simulink model "LQR_spring_2mass_damper_system"  (R2022b)
settings: Solver=FixedStepAuto  StartTime=0  StopTime=Tf  FixedStep=dt  RelTol=1e-3
values from neighbouring files (symbols this model uses):
  A = [0 1 0 0; -(k1+k2)/m1 -(c1+c2)/m1 k2/m1 c2/m1;0 0 0 1;k2/m2 c2/m2 -k2/m2 -c2/m2]    [LQR_2mass__slx_main.m]
  B = [0 0;1/m1 0;0 0;0 1/m2]    [LQR_2mass__slx_main.m]
  c1 = 1    [LQR_2mass__slx_main.m]
  c2 = 2    [LQR_2mass__slx_main.m]
  control_on = true    [LQR_2mass__slx_main.m]
  control_period = 0.1    [LQR_2mass__slx_main.m]
  K = inv(R)*B'*P    [LQR_2mass__slx_main.m]
  k1 = 10    [LQR_2mass__slx_main.m]
  k2 = 20    [LQR_2mass__slx_main.m]
  m1 = 1    [LQR_2mass__slx_main.m]
  m2 = 5    [LQR_2mass__slx_main.m]
  r = [0 0 0 0]'    [LQR_2mass__slx_main.m]
  v1 = 0    [LQR_2mass__slx_main.m]
  v2 = 0    [LQR_2mass__slx_main.m]
  x1 = 1    [LQR_2mass__slx_main.m]
  x2 = 2    [LQR_2mass__slx_main.m]
settings Model: Creator=murayama  LastModifiedBy=murayama
settings DataIOCC: SaveFormat=StructureWithTime  ReturnWorkspaceOutputs=off
settings OptimizationCC: BlockReduction=off  BufferReuse=off
settings DebuggingCC: AlgebraicLoopMsg=none

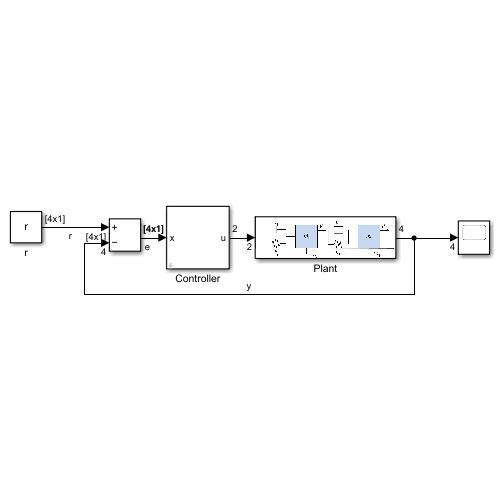
[thumbnail: Simulink's stored preview of the top-level diagram]
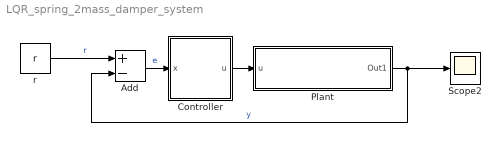
== system LQR_spring_2mass_damper_system ==
  Add : Sum  Inputs=+-
  Controller : Subsystem  mask{LQR=0}
      mask DialogControl ParameterGroupVar Prompt: パラメーター
  Plant : Subsystem
      mask Display: image('C:\Users\murayama\Pictures\バネマスダンパ.png'); % 変更するには、ツールストリップの [イメージの編集] を使用してください。
  Scope2 : Scope
  r : Constant  Value=r  VectorParams1D=off
  wires:
  Plant/1(Out1) -> Scope2/1, Add/2  "y"
  r/1 -> Add/1  "r"
  Add/1 -> Controller/1(x)  "e"
  Controller/1(u) -> Plant/1(u)

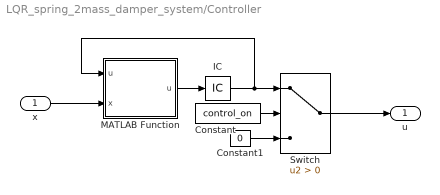
== system LQR_spring_2mass_damper_system/Controller ==
  x : Inport
  Constant : Constant  Value=control_on
  Constant1 : Constant  Value=0
  IC : InitialCondition  Value=[0 0]'
  MATLAB Function : MATLAB Function  TreatAsAtomicUnit=on
  Switch : Switch  Criteria=u2 > Threshold  SaturateOnIntegerOverflow=off  InputSameDT=off
  u : Outport
  wires:
  x/1 -> MATLAB Function/2(x)
  Switch/1 -> u/1
  Constant/1 -> Switch/2
  Constant1/1 -> Switch/3
  MATLAB Function/1(u) -> IC/1
  IC/1 -> MATLAB Function/1("u "), Switch/1

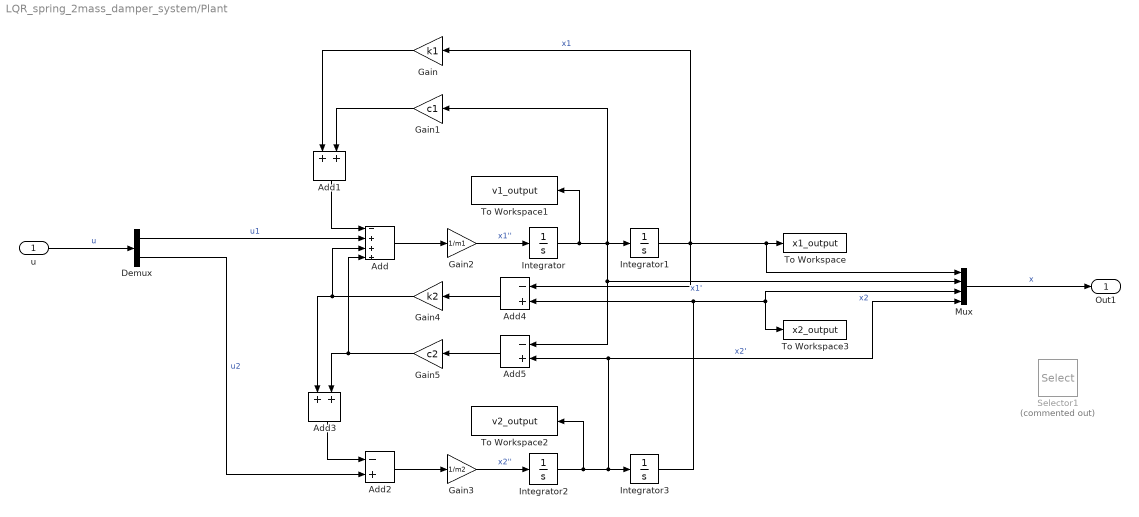
== system LQR_spring_2mass_damper_system/Plant ==
  u : Inport
  Add : Sum  Inputs=-+++
  Add1 : Sum
  Add2 : Sum  Inputs=-+
  Add3 : Sum
  Add4 : Sum  Inputs=-+
  Add5 : Sum  Inputs=-+
  Demux : Demux  Outputs=2
  Gain : Gain  Gain=k1
  Gain1 : Gain  Gain=c1
  Gain2 : Gain  Gain=1/m1
  Gain3 : Gain  Gain=1/m2
  Gain4 : Gain  Gain=k2
  Gain5 : Gain  Gain=c2
  Integrator : Integrator  InitialCondition=v1
  Integrator1 : Integrator  InitialCondition=x1
  Integrator2 : Integrator  InitialCondition=v2
  Integrator3 : Integrator  InitialCondition=x2
  Mux : Mux
  Selector1 : Selector  Commented=on  InputPortWidth=4  IndexOptions=Index vector (dialog)  Indices=[1 3]  OutputSizes=1
  To Workspace : ToWorkspace  VariableName=x1_output  SaveFormat=Timeseries  SampleTime=-1
  To Workspace1 : ToWorkspace  VariableName=v1_output  SaveFormat=Timeseries  SampleTime=-1
  To Workspace2 : ToWorkspace  VariableName=v2_output  SaveFormat=Timeseries  SampleTime=-1
  To Workspace3 : ToWorkspace  VariableName=x2_output  SaveFormat=Timeseries  SampleTime=-1
  Out1 : Outport
  wires:
  Integrator1/1 -> To Workspace/1, Mux/1, Gain/1, Add4/1  "x1"
  Add1/1 -> Add/1
  Gain/1 -> Add1/1
  Add/1 -> Gain2/1
  Gain2/1 -> Integrator/1  "x1''"
  Integrator/1 -> Add5/1, Mux/2, Gain1/1, Integrator1/1, To Workspace1/1  "x1'"
  Gain1/1 -> Add1/2
  Add2/1 -> Gain3/1
  Gain3/1 -> Integrator2/1  "x2''"
  Integrator2/1 -> To Workspace2/1, Mux/4, Add5/2, Integrator3/1  "x2'"
  Integrator3/1 -> Mux/3, To Workspace3/1, Add4/2  "x2"
  Gain4/1 -> Add3/1, Add/3
  Gain5/1 -> Add/4, Add3/2
  Add3/1 -> Add2/1
  Add4/1 -> Gain4/1
  Add5/1 -> Gain5/1
  Mux/1 -> Out1/1  "x"
  Demux/2 -> Add2/2  "u2"
  Demux/1 -> Add/2  "u1"
  u/1 -> Demux/1  "u"

== matlab function LQR_spring_2mass_damper_system/Controller/MATLAB Function ==
  data: u input; x input; u output; K parameter; A parameter; B parameter; control_period parameter
function u = fcn(u,x, K, A, B, control_period)
%% 4th Runge-Kutta method
dt = control_period; %control_period
x
x1 = x;        b1 = dt*(A*x1+B*u);
x2 = x+b1/2;   b2 = dt*(A*x2+B*u);
x3 = x+b2/2;   b3 = dt*(A*x3+B*u);
x4 = x+b3;     b4 = dt*(A*x4+B*u);
x = x+(b1+2*b2+2*b3+b4)/6;
u = K*x;
end
